simulink model "mcb_pmsm_foc_hall_f28035"  (R2021b)
settings: Solver=FixedStepDiscrete  StartTime=0.0  StopTime=8  RelTol=1e-3  EnableMultiTasking=on
InitFcn:
  | mcb_pmsm_foc_hall_f28035_data
values from neighbouring files (symbols this model uses):
  inverter = mcb_SetInverterParameters('BoostXL-DRV8305')    [mcb_pmsm_foc_dual_f28379d_data.m]    (also in mcb_pmsm_foc_dual_f28379d_datascript.m; mcb_pmsm_foc_f280049C_data.m; mcb_pmsm_foc_f28335_data.m = mcb_SetInverterParameters('DRV8312-C2-KIT'); mcb_pmsm_foc_hall_f28035_data.m = mcb_SetInverterParameters('DRV8312-C2-KIT'))
  PI_params = mcb.internal.SetControllerParameters(pmsm,inverter,PU_System,T_pwm,2*Ts,Ts_speed)    [mcb_pmsm_foc_dual_f28379d_data.m]    (also in mcb_pmsm_foc_dual_f28379d_datascript.m; mcb_pmsm_foc_f280049C_data.m = mcb.internal.SetControllerParameters(pmsm,inverter,PU_System; mcb_pmsm_foc_f28335_data.m = mcb.internal.SetControllerParameters(pmsm,inverter,PU_System; mcb_pmsm_foc_hall_f28035_data.m = mcb.internal.SetControllerParameters(pmsm,inverter,PU_System)
  pmsm = struct    [c28335_pmsmfoc_data.m]    (also in mcb_pmsm_foc_dual_f28379d_data.m = mcb_SetPMSMMotorParameters('Teknic2310P'); mcb_pmsm_foc_dual_f28379d_datascript.m = mcb_SetPMSMMotorParameters('Teknic2310P'); mcb_pmsm_foc_f280049C_data.m = mcb_SetPMSMMotorParameters('BLY171D'); mcb_pmsm_foc_f28335_data.m = mcb_SetPMSMMotorParameters('BLY171D'))
  target = mcb_SetProcessorDetails('F28379D',PWM_frequency)    [mcb_pmsm_foc_dual_f28379d_data.m]    (also in mcb_pmsm_foc_dual_f28379d_datascript.m; mcb_pmsm_foc_f280049C_data.m = mcb_SetProcessorDetails('F280049C',PWM_frequency); mcb_pmsm_foc_f28335_data.m = mcb_SetProcessorDetails('F28335',PWM_frequency); mcb_pmsm_foc_hall_f28035_data.m = mcb_SetProcessorDetails('F28035',PWM_frequency))
  Ts = 5e-8    (= 5e-08)    [DCDC_Buck_Param.m]    (also in mcb_c2000_open_loop_control_data.m = T_pwm; mcb_c2000_pmsm_offset_data.m = T_pwm; mcb_pmsm_foc_dual_f28379d_data.m = 5e-05; mcb_pmsm_foc_dual_f28379d_datascript.m = 5e-05)
  Ts_motor = T_pwm/2    (= 2.5e-05)    [mcb_pmsm_foc_dual_f28379d_data.m]    (also in mcb_pmsm_foc_dual_f28379d_datascript.m; mcb_pmsm_foc_f280049C_data.m; mcb_pmsm_foc_f28335_data.m; mcb_pmsm_foc_hall_f28035_data.m)
  Ts_simulink = T_pwm/2    (= 2.5e-05)    [mcb_pmsm_foc_dual_f28379d_data.m]    (also in mcb_pmsm_foc_dual_f28379d_datascript.m; mcb_pmsm_foc_f280049C_data.m; mcb_pmsm_foc_f28335_data.m; mcb_pmsm_foc_hall_f28035_data.m)
undefined symbols (not defined in the file or in its folder): Down, GPTRIP1SEL, GPTRIP2SEL, TZ1, TZ2, Up
libraries: simulink x16, idelinklib_common x15, mcbpositiondecoderlib x7, c2802xlib x5, mcbcontrolslib x3, c280xlib x3, hall_sensor_lib x3, c2803xlib x3, svdutilitieslib x2, demo_controls x1, c2000lib x1, mcbplantlib x1
(part 3 of 3)

== system mcb_pmsm_foc_hall_f28035/Embedded Processor/Hall Algorithm/Input Scaling/Read_Sensor (codegen)/Calculate Position from Hall/Atomic Hall Reading/Function-Call Subsystem1/Direction 0 Provides offset and counter values ==
  halls : Inport
  Action Port : ActionPort  ActionPortLabel=if(u1 == 1)
  Hall A falling : Subsystem  TreatAsAtomicUnit=on
  Hall A rising : Subsystem  TreatAsAtomicUnit=on
  Hall B falling : Subsystem  TreatAsAtomicUnit=on
  Hall B rising : Subsystem  TreatAsAtomicUnit=on
  Hall C falling : Subsystem  TreatAsAtomicUnit=on
  Hall C rising : Subsystem  TreatAsAtomicUnit=on
  Merge : Merge  Inputs=6
  Signal Conversion : SignalConversion  OverrideOpt=on
  Switch Case : SwitchCase  CaseConditions={1,2,3,4,5,6}  ShowDefaultCase=off
  counter : Outport
  wires:
  Signal Conversion/1 -> counter/1
  Hall B rising/1(counter) -> Merge/6
  Hall C rising/1(counter) -> Merge/5
  Hall A falling/1(counter) -> Merge/4
  Hall A rising/1(counter) -> Merge/3
  Hall C falling/1(counter) -> Merge/2
  Hall B falling/1(counter) -> Merge/1
  Merge/1 -> Signal Conversion/1
  Switch Case/4 -> Hall A falling/Action
  Switch Case/3 -> Hall A rising/Action
  Switch Case/1 -> Hall B falling/Action
  Switch Case/6 -> Hall B rising/Action
  Switch Case/5 -> Hall C rising/Action
  Switch Case/2 -> Hall C falling/Action
  halls/1 -> Switch Case/1

== system mcb_pmsm_foc_hall_f28035/Embedded Processor/Hall Algorithm/Input Scaling/Read_Sensor (codegen)/Calculate Position from Hall/Atomic Hall Reading/Function-Call Subsystem1/Direction 1 Provides offset and counter values ==
  halls : Inport
  Action Port : ActionPort  ActionPortLabel=else
  Hall A falling : Subsystem  TreatAsAtomicUnit=on
  Hall A rising : Subsystem  TreatAsAtomicUnit=on
  Hall B falling : Subsystem  TreatAsAtomicUnit=on
  Hall B rising : Subsystem  TreatAsAtomicUnit=on
  Hall C falling : Subsystem  TreatAsAtomicUnit=on
  Hall C rising : Subsystem  TreatAsAtomicUnit=on
  Merge : Merge  Inputs=6
  Switch Case : SwitchCase  CaseConditions={1,2,3,4,5,6}  ShowDefaultCase=off
  counter : Outport
  wires:
  Hall C rising/1(counter) -> Merge/6
  Hall A rising/1(counter) -> Merge/5
  Hall B falling/1(counter) -> Merge/4
  Hall B rising/1(counter) -> Merge/3
  Hall A falling/1(counter) -> Merge/2
  Hall C falling/1(counter) -> Merge/1
  Switch Case/4 -> Hall B falling/Action
  Switch Case/3 -> Hall B rising/Action
  Switch Case/1 -> Hall C falling/Action
  Switch Case/6 -> Hall C rising/Action
  Switch Case/5 -> Hall A rising/Action
  Switch Case/2 -> Hall A falling/Action
  halls/1 -> Switch Case/1
  Merge/1 -> counter/1

== system mcb_pmsm_foc_hall_f28035/Embedded Processor/Hall Algorithm/Input Scaling/Read_Sensor (codegen)/Calculate Position from Hall/Atomic Hall Reading/Function-Call Subsystem4/Direction 0 Provides offset and counter values ==
  halls : Inport
  In2 : Inport  Port=2
  Action Port : ActionPort  ActionPortLabel=if(u1 == 1)
  Hall A falling : Subsystem  TreatAsAtomicUnit=on
  Hall A rising : Subsystem  TreatAsAtomicUnit=on
  Hall B falling : Subsystem  TreatAsAtomicUnit=on
  Hall B rising : Subsystem  TreatAsAtomicUnit=on
  Hall C falling : Subsystem  TreatAsAtomicUnit=on
  Hall C rising : Subsystem  TreatAsAtomicUnit=on
  Merge : Merge  Inputs=6
  Signal Conversion : SignalConversion  OverrideOpt=on
  Switch Case : SwitchCase  CaseConditions={1,2,3,4,5,6}  ShowDefaultCase=off
  counter : Outport
  wires:
  In2/1 -> Hall B falling/1(In1), Hall C falling/1(In1), Hall A rising/1(In1), Hall A falling/1(In1), Hall C rising/1(In1), Hall B rising/1(In1)
  Signal Conversion/1 -> counter/1
  Hall B rising/1(counter) -> Merge/6
  Hall C rising/1(counter) -> Merge/5
  Hall A falling/1(counter) -> Merge/4
  Hall A rising/1(counter) -> Merge/3
  Hall C falling/1(counter) -> Merge/2
  Hall B falling/1(counter) -> Merge/1
  Merge/1 -> Signal Conversion/1
  Switch Case/4 -> Hall A falling/Action
  Switch Case/3 -> Hall A rising/Action
  Switch Case/1 -> Hall B falling/Action
  Switch Case/6 -> Hall B rising/Action
  Switch Case/5 -> Hall C rising/Action
  Switch Case/2 -> Hall C falling/Action
  halls/1 -> Switch Case/1

== system mcb_pmsm_foc_hall_f28035/Embedded Processor/Hall Algorithm/Input Scaling/Read_Sensor (codegen)/Calculate Position from Hall/Atomic Hall Reading/Function-Call Subsystem4/Direction 1 Provides offset and counter values ==
  In1 : Inport
  halls : Inport  Port=2
  Action Port : ActionPort  ActionPortLabel=else
  Hall A falling : Subsystem  TreatAsAtomicUnit=on
  Hall A rising : Subsystem  TreatAsAtomicUnit=on
  Hall B falling : Subsystem  TreatAsAtomicUnit=on
  Hall B rising : Subsystem  TreatAsAtomicUnit=on
  Hall C falling : Subsystem  TreatAsAtomicUnit=on
  Hall C rising : Subsystem  TreatAsAtomicUnit=on
  Merge : Merge  Inputs=6
  Switch Case : SwitchCase  CaseConditions={1,2,3,4,5,6}  ShowDefaultCase=off
  counter : Outport
  wires:
  In1/1 -> Hall C falling/1(In1), Hall A falling/1(In1), Hall B rising/1(In1), Hall B falling/1(In1), Hall A rising/1(In1), Hall C rising/1(In1)
  Hall C rising/1(counter) -> Merge/6
  Hall A rising/1(counter) -> Merge/5
  Hall B falling/1(counter) -> Merge/4
  Hall B rising/1(counter) -> Merge/3
  Hall A falling/1(counter) -> Merge/2
  Hall C falling/1(counter) -> Merge/1
  Switch Case/4 -> Hall B falling/Action
  Switch Case/3 -> Hall B rising/Action
  Switch Case/1 -> Hall C falling/Action
  Switch Case/6 -> Hall C rising/Action
  Switch Case/5 -> Hall A rising/Action
  Switch Case/2 -> Hall A falling/Action
  halls/1 -> Switch Case/1
  Merge/1 -> counter/1

== system mcb_pmsm_foc_hall_f28035/Embedded Processor/Hall Algorithm/Input Scaling/Read_Sensor (codegen)/Calculate Position from Hall/Atomic Hall Reading/Function-Call Subsystem/Integrity_Check/No_Integrity_issue ==
  Counter : Inport
  Action Port : ActionPort  ActionPortLabel=if(u1 == 0)
  Out1 : Outport
  wires:
  Counter/1 -> Out1/1

== system mcb_pmsm_foc_hall_f28035/Embedded Processor/Hall Algorithm/Input Scaling/Read_Sensor (codegen)/Calculate Position from Hall/Atomic Hall Reading/Function-Call Subsystem/Integrity_Check/Refresh_Halls ==
  Action Port : ActionPort  ActionPortLabel=else
  Bitwise AND : simulink/Logic and Bit Operations/Bitwise Operator  logicop=AND  UseBitMask=on  BitMask=hex2dec('07000000')  BitMaskRealWorld=Stored Integer
  Data Type Conversion : DataTypeConversion  OutDataTypeStr=uint32  ConvertRealWorld=Stored Integer (SI)
  Memory Copy3 : svdutilitieslib/Memory Copy  copyFrom=Specified source code symbol  copyFromAddressSource=Specify via dialog  copyFromAddress=hex2dec('00001000')  copyFromSrcCode=&GpioDataRegs.GPADAT.all  dataTypeFrom=uint32  dataDimensionFrom=1  useOffsetFrom=off  offsetFromSrc=Specify via dialog  offsetFrom=0  strideFrom=1  copyTo=Output port  copyToAddressSource=Specify via dialog  copyToAddress=hex2dec('00002000')  copyToSrcCode=myVariableDst  dataTypeTo=uint32  useOffsetTo=off  offsetToSrc=Specify via dialog  offsetTo=0  strideTo=1  sampleTime=-1  useInitValue=off  initValueSrc=Specify constant value  initValue=1  initValueSrcCode=myInitValueVariable  useAsMask=off  maskOperator=bitwise AND  useTermValue=off  termValue=1  isRealtimeEnabled=off  emitCCBeforeWrite=off  CCBeforeWrite=/* Custom Code Before Write*/  emitCCAfterWrite=off  CCAfterWrite=/* Custom Code After Write*/  useDMACopy=off  enableBlockingMode=off  blockPlatform=arduinoert
      settings: SourceProductBaseCode=ANDROID,ARDUINO,ML_ARDUINO,ECCORTEXA,ECCORTEXR,SC_BEAGLEBONE_BLUE,EC_FREEDOM_BOARD,EC_FRDM_K64F,INTEL_BLOCKSET,MICROBIT,NUCLEO,NVIDIA,PX4AUTOPILOTS,RASPPIIO,STMICRODIS,TIC2000,XILINX_BLOCKSET
  Shift Arithmetic : ArithShift  BitShiftNumber=24
  Out1 : Outport
  wires:
  Data Type Conversion/1 -> Out1/1
  Bitwise AND/1 -> Shift Arithmetic/1
  Shift Arithmetic/1 -> Data Type Conversion/1
  Memory Copy3/1 -> Bitwise AND/1

== system mcb_pmsm_foc_hall_f28035/Embedded Processor/Hall Algorithm/Input Scaling/Read_Sensor (codegen)/Calculate Position from Hall/Atomic Hall Reading/Function-Call Subsystem1/Direction 0 Provides offset and counter values/Hall A falling ==
  Action Port : ActionPort  ActionPortLabel=case [ 4 ]:
  ECap1Regs.TSCTR1 : idelinklib_common/Memory Copy  copyFrom=Specified source code symbol  copyFromAddressSource=Specify via dialog  copyFromAddress=hex2dec('00001000')  copyFromSrcCode=&ECap1Regs.TSCTR  dataTypeFrom=uint32  dataDimensionFrom=1  useOffsetFrom=off  offsetFromSrc=Specify via dialog  offsetFrom=0  strideFrom=1  copyTo=Output port  copyToAddressSource=Specify via dialog  copyToAddress=hex2dec('00002000')  copyToSrcCode=myVariableDst  dataTypeTo=uint32  useOffsetTo=off  offsetToSrc=Specify via dialog  offsetTo=0  strideTo=1  sampleTime=-1  useInitValue=off  initValueSrc=Specify constant value  initValue=1  initValueSrcCode=myInitValueVariable  useAsMask=off  maskOperator=bitwise AND  useTermValue=off  termValue=1  isRealtimeEnabled=off  emitCCBeforeWrite=off  CCBeforeWrite=/* Custom Code Before Write*/  emitCCAfterWrite=off  CCAfterWrite=/* Custom Code After Write*/  useDMACopy=off  enableBlockingMode=off
      settings: SourceProductBaseCode=ME
  counter : Outport
  wires:
  ECap1Regs.TSCTR1/1 -> counter/1

== system mcb_pmsm_foc_hall_f28035/Embedded Processor/Hall Algorithm/Input Scaling/Read_Sensor (codegen)/Calculate Position from Hall/Atomic Hall Reading/Function-Call Subsystem1/Direction 0 Provides offset and counter values/Hall A rising ==
  Action Port : ActionPort  ActionPortLabel=case [ 3 ]:
  ECap1Regs.TSCTR1 : idelinklib_common/Memory Copy  copyFrom=Specified source code symbol  copyFromAddressSource=Specify via dialog  copyFromAddress=hex2dec('00001000')  copyFromSrcCode=&ECap1Regs.TSCTR  dataTypeFrom=uint32  dataDimensionFrom=1  useOffsetFrom=off  offsetFromSrc=Specify via dialog  offsetFrom=0  strideFrom=1  copyTo=Output port  copyToAddressSource=Specify via dialog  copyToAddress=hex2dec('00002000')  copyToSrcCode=myVariableDst  dataTypeTo=uint32  useOffsetTo=off  offsetToSrc=Specify via dialog  offsetTo=0  strideTo=1  sampleTime=-1  useInitValue=off  initValueSrc=Specify constant value  initValue=1  initValueSrcCode=myInitValueVariable  useAsMask=off  maskOperator=bitwise AND  useTermValue=off  termValue=1  isRealtimeEnabled=off  emitCCBeforeWrite=off  CCBeforeWrite=/* Custom Code Before Write*/  emitCCAfterWrite=off  CCAfterWrite=/* Custom Code After Write*/  useDMACopy=off  enableBlockingMode=off
      settings: SourceProductBaseCode=ME
  counter : Outport
  wires:
  ECap1Regs.TSCTR1/1 -> counter/1

== system mcb_pmsm_foc_hall_f28035/Embedded Processor/Hall Algorithm/Input Scaling/Read_Sensor (codegen)/Calculate Position from Hall/Atomic Hall Reading/Function-Call Subsystem1/Direction 0 Provides offset and counter values/Hall B falling ==
  Action Port : ActionPort  ActionPortLabel=case [ 1 ]:
  Add : Sum  Inputs=-+  OutDataTypeStr=Inherit: Same as first input
  Data Store Read : DataStoreRead  DataStoreName=ECap1_counter_XINT1_latch  IndexOptions=Index vector (dialog)  Indices=1  OutputSizes=1
  ECap1Regs.TSCTR : idelinklib_common/Memory Copy  copyFrom=Specified source code symbol  copyFromAddressSource=Specify via dialog  copyFromAddress=hex2dec('00001000')  copyFromSrcCode=&ECap1Regs.TSCTR  dataTypeFrom=uint32  dataDimensionFrom=1  useOffsetFrom=off  offsetFromSrc=Specify via dialog  offsetFrom=0  strideFrom=1  copyTo=Output port  copyToAddressSource=Specify via dialog  copyToAddress=hex2dec('00002000')  copyToSrcCode=myVariableDst  dataTypeTo=uint32  useOffsetTo=off  offsetToSrc=Specify via dialog  offsetTo=0  strideTo=1  sampleTime=-1  useInitValue=off  initValueSrc=Specify constant value  initValue=1  initValueSrcCode=myInitValueVariable  useAsMask=off  maskOperator=bitwise AND  useTermValue=off  termValue=1  isRealtimeEnabled=off  emitCCBeforeWrite=off  CCBeforeWrite=/* Custom Code Before Write*/  emitCCAfterWrite=off  CCAfterWrite=/* Custom Code After Write*/  useDMACopy=off  enableBlockingMode=off
      settings: SourceProductBaseCode=ME
  counter : Outport
  wires:
  Add/1 -> counter/1
  ECap1Regs.TSCTR/1 -> Add/2
  Data Store Read/1 -> Add/1

== system mcb_pmsm_foc_hall_f28035/Embedded Processor/Hall Algorithm/Input Scaling/Read_Sensor (codegen)/Calculate Position from Hall/Atomic Hall Reading/Function-Call Subsystem1/Direction 0 Provides offset and counter values/Hall B rising ==
  Action Port : ActionPort  ActionPortLabel=case [ 6 ]:
  Add : Sum  Inputs=-+  OutDataTypeStr=Inherit: Same as first input
  Data Store Read : DataStoreRead  DataStoreName=ECap1_counter_XINT1_latch  IndexOptions=Index vector (dialog)  Indices=1  OutputSizes=1
  ECap1Regs.TSCTR : idelinklib_common/Memory Copy  copyFrom=Specified source code symbol  copyFromAddressSource=Specify via dialog  copyFromAddress=hex2dec('00001000')  copyFromSrcCode=&ECap1Regs.TSCTR  dataTypeFrom=uint32  dataDimensionFrom=1  useOffsetFrom=off  offsetFromSrc=Specify via dialog  offsetFrom=0  strideFrom=1  copyTo=Output port  copyToAddressSource=Specify via dialog  copyToAddress=hex2dec('00002000')  copyToSrcCode=myVariableDst  dataTypeTo=uint32  useOffsetTo=off  offsetToSrc=Specify via dialog  offsetTo=0  strideTo=1  sampleTime=-1  useInitValue=off  initValueSrc=Specify constant value  initValue=1  initValueSrcCode=myInitValueVariable  useAsMask=off  maskOperator=bitwise AND  useTermValue=off  termValue=1  isRealtimeEnabled=off  emitCCBeforeWrite=off  CCBeforeWrite=/* Custom Code Before Write*/  emitCCAfterWrite=off  CCAfterWrite=/* Custom Code After Write*/  useDMACopy=off  enableBlockingMode=off
      settings: SourceProductBaseCode=ME
  counter : Outport
  wires:
  ECap1Regs.TSCTR/1 -> Add/2
  Data Store Read/1 -> Add/1
  Add/1 -> counter/1

== system mcb_pmsm_foc_hall_f28035/Embedded Processor/Hall Algorithm/Input Scaling/Read_Sensor (codegen)/Calculate Position from Hall/Atomic Hall Reading/Function-Call Subsystem1/Direction 0 Provides offset and counter values/Hall C falling ==
  Action Port : ActionPort  ActionPortLabel=case [ 2 ]:
  Add : Sum  Inputs=-+  OutDataTypeStr=Inherit: Same as first input
  Data Store Read : DataStoreRead  DataStoreName=ECap1_counter_XINT2_latch  IndexOptions=Index vector (dialog)  Indices=1  OutputSizes=1
  ECap1Regs.TSCTR : idelinklib_common/Memory Copy  copyFrom=Specified source code symbol  copyFromAddressSource=Specify via dialog  copyFromAddress=hex2dec('00001000')  copyFromSrcCode=&ECap1Regs.TSCTR  dataTypeFrom=uint32  dataDimensionFrom=1  useOffsetFrom=off  offsetFromSrc=Specify via dialog  offsetFrom=0  strideFrom=1  copyTo=Output port  copyToAddressSource=Specify via dialog  copyToAddress=hex2dec('00002000')  copyToSrcCode=myVariableDst  dataTypeTo=uint32  useOffsetTo=off  offsetToSrc=Specify via dialog  offsetTo=0  strideTo=1  sampleTime=-1  useInitValue=off  initValueSrc=Specify constant value  initValue=1  initValueSrcCode=myInitValueVariable  useAsMask=off  maskOperator=bitwise AND  useTermValue=off  termValue=1  isRealtimeEnabled=off  emitCCBeforeWrite=off  CCBeforeWrite=/* Custom Code Before Write*/  emitCCAfterWrite=off  CCAfterWrite=/* Custom Code After Write*/  useDMACopy=off  enableBlockingMode=off
      settings: SourceProductBaseCode=ME
  counter : Outport
  wires:
  ECap1Regs.TSCTR/1 -> Add/2
  Data Store Read/1 -> Add/1
  Add/1 -> counter/1

== system mcb_pmsm_foc_hall_f28035/Embedded Processor/Hall Algorithm/Input Scaling/Read_Sensor (codegen)/Calculate Position from Hall/Atomic Hall Reading/Function-Call Subsystem1/Direction 0 Provides offset and counter values/Hall C rising ==
  Action Port : ActionPort  ActionPortLabel=case [ 5 ]:
  Add : Sum  Inputs=-+  OutDataTypeStr=Inherit: Same as first input
  Data Store Read : DataStoreRead  DataStoreName=ECap1_counter_XINT2_latch  IndexOptions=Index vector (dialog)  Indices=1  OutputSizes=1
  ECap1Regs.TSCTR : idelinklib_common/Memory Copy  copyFrom=Specified source code symbol  copyFromAddressSource=Specify via dialog  copyFromAddress=hex2dec('00001000')  copyFromSrcCode=&ECap1Regs.TSCTR  dataTypeFrom=uint32  dataDimensionFrom=1  useOffsetFrom=off  offsetFromSrc=Specify via dialog  offsetFrom=0  strideFrom=1  copyTo=Output port  copyToAddressSource=Specify via dialog  copyToAddress=hex2dec('00002000')  copyToSrcCode=myVariableDst  dataTypeTo=uint32  useOffsetTo=off  offsetToSrc=Specify via dialog  offsetTo=0  strideTo=1  sampleTime=-1  useInitValue=off  initValueSrc=Specify constant value  initValue=1  initValueSrcCode=myInitValueVariable  useAsMask=off  maskOperator=bitwise AND  useTermValue=off  termValue=1  isRealtimeEnabled=off  emitCCBeforeWrite=off  CCBeforeWrite=/* Custom Code Before Write*/  emitCCAfterWrite=off  CCAfterWrite=/* Custom Code After Write*/  useDMACopy=off  enableBlockingMode=off
      settings: SourceProductBaseCode=ME
  counter : Outport
  wires:
  ECap1Regs.TSCTR/1 -> Add/2
  Data Store Read/1 -> Add/1
  Add/1 -> counter/1

== system mcb_pmsm_foc_hall_f28035/Embedded Processor/Hall Algorithm/Input Scaling/Read_Sensor (codegen)/Calculate Position from Hall/Atomic Hall Reading/Function-Call Subsystem1/Direction 1 Provides offset and counter values/Hall A falling ==
  Action Port : ActionPort  ActionPortLabel=case [ 2 ]:
  ECap1Regs.TSCTR1 : idelinklib_common/Memory Copy  copyFrom=Specified source code symbol  copyFromAddressSource=Specify via dialog  copyFromAddress=hex2dec('00001000')  copyFromSrcCode=&ECap1Regs.TSCTR  dataTypeFrom=uint32  dataDimensionFrom=1  useOffsetFrom=off  offsetFromSrc=Specify via dialog  offsetFrom=0  strideFrom=1  copyTo=Output port  copyToAddressSource=Specify via dialog  copyToAddress=hex2dec('00002000')  copyToSrcCode=myVariableDst  dataTypeTo=uint32  useOffsetTo=off  offsetToSrc=Specify via dialog  offsetTo=0  strideTo=1  sampleTime=-1  useInitValue=off  initValueSrc=Specify constant value  initValue=1  initValueSrcCode=myInitValueVariable  useAsMask=off  maskOperator=bitwise AND  useTermValue=off  termValue=1  isRealtimeEnabled=off  emitCCBeforeWrite=off  CCBeforeWrite=/* Custom Code Before Write*/  emitCCAfterWrite=off  CCAfterWrite=/* Custom Code After Write*/  useDMACopy=off  enableBlockingMode=off
      settings: SourceProductBaseCode=ME
  counter : Outport
  wires:
  ECap1Regs.TSCTR1/1 -> counter/1

== system mcb_pmsm_foc_hall_f28035/Embedded Processor/Hall Algorithm/Input Scaling/Read_Sensor (codegen)/Calculate Position from Hall/Atomic Hall Reading/Function-Call Subsystem1/Direction 1 Provides offset and counter values/Hall A rising ==
  Action Port : ActionPort  ActionPortLabel=case [ 5 ]:
  ECap1Regs.TSCTR1 : idelinklib_common/Memory Copy  copyFrom=Specified source code symbol  copyFromAddressSource=Specify via dialog  copyFromAddress=hex2dec('00001000')  copyFromSrcCode=&ECap1Regs.TSCTR  dataTypeFrom=uint32  dataDimensionFrom=1  useOffsetFrom=off  offsetFromSrc=Specify via dialog  offsetFrom=0  strideFrom=1  copyTo=Output port  copyToAddressSource=Specify via dialog  copyToAddress=hex2dec('00002000')  copyToSrcCode=myVariableDst  dataTypeTo=uint32  useOffsetTo=off  offsetToSrc=Specify via dialog  offsetTo=0  strideTo=1  sampleTime=-1  useInitValue=off  initValueSrc=Specify constant value  initValue=1  initValueSrcCode=myInitValueVariable  useAsMask=off  maskOperator=bitwise AND  useTermValue=off  termValue=1  isRealtimeEnabled=off  emitCCBeforeWrite=off  CCBeforeWrite=/* Custom Code Before Write*/  emitCCAfterWrite=off  CCAfterWrite=/* Custom Code After Write*/  useDMACopy=off  enableBlockingMode=off
      settings: SourceProductBaseCode=ME
  counter : Outport
  wires:
  ECap1Regs.TSCTR1/1 -> counter/1

== system mcb_pmsm_foc_hall_f28035/Embedded Processor/Hall Algorithm/Input Scaling/Read_Sensor (codegen)/Calculate Position from Hall/Atomic Hall Reading/Function-Call Subsystem1/Direction 1 Provides offset and counter values/Hall B falling ==
  Action Port : ActionPort  ActionPortLabel=case [ 4 ]:
  Add : Sum  Inputs=+-  OutDataTypeStr=Inherit: Same as first input
  Data Store Read : DataStoreRead  DataStoreName=ECap1_counter_XINT1_latch  IndexOptions=Index vector (dialog)  Indices=1  OutputSizes=1
  ECap1Regs.TSCTR : idelinklib_common/Memory Copy  copyFrom=Specified source code symbol  copyFromAddressSource=Specify via dialog  copyFromAddress=hex2dec('00001000')  copyFromSrcCode=&ECap1Regs.TSCTR  dataTypeFrom=uint32  dataDimensionFrom=1  useOffsetFrom=off  offsetFromSrc=Specify via dialog  offsetFrom=0  strideFrom=1  copyTo=Output port  copyToAddressSource=Specify via dialog  copyToAddress=hex2dec('00002000')  copyToSrcCode=myVariableDst  dataTypeTo=uint32  useOffsetTo=off  offsetToSrc=Specify via dialog  offsetTo=0  strideTo=1  sampleTime=-1  useInitValue=off  initValueSrc=Specify constant value  initValue=1  initValueSrcCode=myInitValueVariable  useAsMask=off  maskOperator=bitwise AND  useTermValue=off  termValue=1  isRealtimeEnabled=off  emitCCBeforeWrite=off  CCBeforeWrite=/* Custom Code Before Write*/  emitCCAfterWrite=off  CCAfterWrite=/* Custom Code After Write*/  useDMACopy=off  enableBlockingMode=off
      settings: SourceProductBaseCode=ME
  counter : Outport
  wires:
  ECap1Regs.TSCTR/1 -> Add/1
  Data Store Read/1 -> Add/2
  Add/1 -> counter/1

== system mcb_pmsm_foc_hall_f28035/Embedded Processor/Hall Algorithm/Input Scaling/Read_Sensor (codegen)/Calculate Position from Hall/Atomic Hall Reading/Function-Call Subsystem1/Direction 1 Provides offset and counter values/Hall B rising ==
  Action Port : ActionPort  ActionPortLabel=case [ 3 ]:
  Add : Sum  Inputs=-+  OutDataTypeStr=Inherit: Same as first input
  Data Store Read : DataStoreRead  DataStoreName=ECap1_counter_XINT1_latch  IndexOptions=Index vector (dialog)  Indices=1  OutputSizes=1
  ECap1Regs.TSCTR : idelinklib_common/Memory Copy  copyFrom=Specified source code symbol  copyFromAddressSource=Specify via dialog  copyFromAddress=hex2dec('00001000')  copyFromSrcCode=&ECap1Regs.TSCTR  dataTypeFrom=uint32  dataDimensionFrom=1  useOffsetFrom=off  offsetFromSrc=Specify via dialog  offsetFrom=0  strideFrom=1  copyTo=Output port  copyToAddressSource=Specify via dialog  copyToAddress=hex2dec('00002000')  copyToSrcCode=myVariableDst  dataTypeTo=uint32  useOffsetTo=off  offsetToSrc=Specify via dialog  offsetTo=0  strideTo=1  sampleTime=-1  useInitValue=off  initValueSrc=Specify constant value  initValue=1  initValueSrcCode=myInitValueVariable  useAsMask=off  maskOperator=bitwise AND  useTermValue=off  termValue=1  isRealtimeEnabled=off  emitCCBeforeWrite=off  CCBeforeWrite=/* Custom Code Before Write*/  emitCCAfterWrite=off  CCAfterWrite=/* Custom Code After Write*/  useDMACopy=off  enableBlockingMode=off
      settings: SourceProductBaseCode=ME
  counter : Outport
  wires:
  ECap1Regs.TSCTR/1 -> Add/2
  Data Store Read/1 -> Add/1
  Add/1 -> counter/1

== system mcb_pmsm_foc_hall_f28035/Embedded Processor/Hall Algorithm/Input Scaling/Read_Sensor (codegen)/Calculate Position from Hall/Atomic Hall Reading/Function-Call Subsystem1/Direction 1 Provides offset and counter values/Hall C falling ==
  Action Port : ActionPort  ActionPortLabel=case [ 1 ]:
  Add : Sum  Inputs=-+  OutDataTypeStr=Inherit: Same as first input
  Data Store Read : DataStoreRead  DataStoreName=ECap1_counter_XINT2_latch  IndexOptions=Index vector (dialog)  Indices=1  OutputSizes=1
  ECap1Regs.TSCTR : idelinklib_common/Memory Copy  copyFrom=Specified source code symbol  copyFromAddressSource=Specify via dialog  copyFromAddress=hex2dec('00001000')  copyFromSrcCode=&ECap1Regs.TSCTR  dataTypeFrom=uint32  dataDimensionFrom=1  useOffsetFrom=off  offsetFromSrc=Specify via dialog  offsetFrom=0  strideFrom=1  copyTo=Output port  copyToAddressSource=Specify via dialog  copyToAddress=hex2dec('00002000')  copyToSrcCode=myVariableDst  dataTypeTo=uint32  useOffsetTo=off  offsetToSrc=Specify via dialog  offsetTo=0  strideTo=1  sampleTime=-1  useInitValue=off  initValueSrc=Specify constant value  initValue=1  initValueSrcCode=myInitValueVariable  useAsMask=off  maskOperator=bitwise AND  useTermValue=off  termValue=1  isRealtimeEnabled=off  emitCCBeforeWrite=off  CCBeforeWrite=/* Custom Code Before Write*/  emitCCAfterWrite=off  CCAfterWrite=/* Custom Code After Write*/  useDMACopy=off  enableBlockingMode=off
      settings: SourceProductBaseCode=ME
  counter : Outport
  wires:
  Data Store Read/1 -> Add/1
  ECap1Regs.TSCTR/1 -> Add/2
  Add/1 -> counter/1

== system mcb_pmsm_foc_hall_f28035/Embedded Processor/Hall Algorithm/Input Scaling/Read_Sensor (codegen)/Calculate Position from Hall/Atomic Hall Reading/Function-Call Subsystem1/Direction 1 Provides offset and counter values/Hall C rising ==
  Action Port : ActionPort  ActionPortLabel=case [ 6 ]:
  Add : Sum  Inputs=-+  OutDataTypeStr=Inherit: Same as first input
  Data Store Read : DataStoreRead  DataStoreName=ECap1_counter_XINT2_latch  IndexOptions=Index vector (dialog)  Indices=1  OutputSizes=1
  ECap1Regs.TSCTR : idelinklib_common/Memory Copy  copyFrom=Specified source code symbol  copyFromAddressSource=Specify via dialog  copyFromAddress=hex2dec('00001000')  copyFromSrcCode=&ECap1Regs.TSCTR  dataTypeFrom=uint32  dataDimensionFrom=1  useOffsetFrom=off  offsetFromSrc=Specify via dialog  offsetFrom=0  strideFrom=1  copyTo=Output port  copyToAddressSource=Specify via dialog  copyToAddress=hex2dec('00002000')  copyToSrcCode=myVariableDst  dataTypeTo=uint32  useOffsetTo=off  offsetToSrc=Specify via dialog  offsetTo=0  strideTo=1  sampleTime=-1  useInitValue=off  initValueSrc=Specify constant value  initValue=1  initValueSrcCode=myInitValueVariable  useAsMask=off  maskOperator=bitwise AND  useTermValue=off  termValue=1  isRealtimeEnabled=off  emitCCBeforeWrite=off  CCBeforeWrite=/* Custom Code Before Write*/  emitCCAfterWrite=off  CCAfterWrite=/* Custom Code After Write*/  useDMACopy=off  enableBlockingMode=off
      settings: SourceProductBaseCode=ME
  counter : Outport
  wires:
  Data Store Read/1 -> Add/1
  ECap1Regs.TSCTR/1 -> Add/2
  Add/1 -> counter/1

== system mcb_pmsm_foc_hall_f28035/Embedded Processor/Hall Algorithm/Input Scaling/Read_Sensor (codegen)/Calculate Position from Hall/Atomic Hall Reading/Function-Call Subsystem4/Direction 0 Provides offset and counter values/Hall A falling ==
  In1 : Inport
  Action Port : ActionPort  ActionPortLabel=case [ 4 ]:
  counter : Outport
  wires:
  In1/1 -> counter/1

== system mcb_pmsm_foc_hall_f28035/Embedded Processor/Hall Algorithm/Input Scaling/Read_Sensor (codegen)/Calculate Position from Hall/Atomic Hall Reading/Function-Call Subsystem4/Direction 0 Provides offset and counter values/Hall A rising ==
  In1 : Inport
  Action Port : ActionPort  ActionPortLabel=case [ 3 ]:
  counter : Outport
  wires:
  In1/1 -> counter/1

== system mcb_pmsm_foc_hall_f28035/Embedded Processor/Hall Algorithm/Input Scaling/Read_Sensor (codegen)/Calculate Position from Hall/Atomic Hall Reading/Function-Call Subsystem4/Direction 0 Provides offset and counter values/Hall B falling ==
  In1 : Inport
  Action Port : ActionPort  ActionPortLabel=case [ 1 ]:
  Add : Sum  Inputs=-+  OutDataTypeStr=Inherit: Same as first input
  Data Store Read : DataStoreRead  DataStoreName=ECap1_counter_XINT1_latch  IndexOptions=Index vector (dialog)  Indices=1  OutputSizes=1
  counter : Outport
  wires:
  Add/1 -> counter/1
  In1/1 -> Add/2
  Data Store Read/1 -> Add/1

== system mcb_pmsm_foc_hall_f28035/Embedded Processor/Hall Algorithm/Input Scaling/Read_Sensor (codegen)/Calculate Position from Hall/Atomic Hall Reading/Function-Call Subsystem4/Direction 0 Provides offset and counter values/Hall B rising ==
  In1 : Inport
  Action Port : ActionPort  ActionPortLabel=case [ 6 ]:
  Add : Sum  Inputs=-+  OutDataTypeStr=Inherit: Same as first input
  Data Store Read : DataStoreRead  DataStoreName=ECap1_counter_XINT1_latch  IndexOptions=Index vector (dialog)  Indices=1  OutputSizes=1
  counter : Outport
  wires:
  In1/1 -> Add/2
  Data Store Read/1 -> Add/1
  Add/1 -> counter/1

== system mcb_pmsm_foc_hall_f28035/Embedded Processor/Hall Algorithm/Input Scaling/Read_Sensor (codegen)/Calculate Position from Hall/Atomic Hall Reading/Function-Call Subsystem4/Direction 0 Provides offset and counter values/Hall C falling ==
  In1 : Inport
  Action Port : ActionPort  ActionPortLabel=case [ 2 ]:
  Add : Sum  Inputs=-+  OutDataTypeStr=Inherit: Same as first input
  Data Store Read : DataStoreRead  DataStoreName=ECap1_counter_XINT2_latch  IndexOptions=Index vector (dialog)  Indices=1  OutputSizes=1
  counter : Outport
  wires:
  In1/1 -> Add/2
  Data Store Read/1 -> Add/1
  Add/1 -> counter/1

== system mcb_pmsm_foc_hall_f28035/Embedded Processor/Hall Algorithm/Input Scaling/Read_Sensor (codegen)/Calculate Position from Hall/Atomic Hall Reading/Function-Call Subsystem4/Direction 0 Provides offset and counter values/Hall C rising ==
  In1 : Inport
  Action Port : ActionPort  ActionPortLabel=case [ 5 ]:
  Add : Sum  Inputs=-+  OutDataTypeStr=Inherit: Same as first input
  Data Store Read : DataStoreRead  DataStoreName=ECap1_counter_XINT2_latch  IndexOptions=Index vector (dialog)  Indices=1  OutputSizes=1
  counter : Outport
  wires:
  In1/1 -> Add/2
  Data Store Read/1 -> Add/1
  Add/1 -> counter/1

== system mcb_pmsm_foc_hall_f28035/Embedded Processor/Hall Algorithm/Input Scaling/Read_Sensor (codegen)/Calculate Position from Hall/Atomic Hall Reading/Function-Call Subsystem4/Direction 1 Provides offset and counter values/Hall A falling ==
  In1 : Inport
  Action Port : ActionPort  ActionPortLabel=case [ 2 ]:
  counter : Outport
  wires:
  In1/1 -> counter/1

== system mcb_pmsm_foc_hall_f28035/Embedded Processor/Hall Algorithm/Input Scaling/Read_Sensor (codegen)/Calculate Position from Hall/Atomic Hall Reading/Function-Call Subsystem4/Direction 1 Provides offset and counter values/Hall A rising ==
  In1 : Inport
  Action Port : ActionPort  ActionPortLabel=case [ 5 ]:
  counter : Outport
  wires:
  In1/1 -> counter/1

== system mcb_pmsm_foc_hall_f28035/Embedded Processor/Hall Algorithm/Input Scaling/Read_Sensor (codegen)/Calculate Position from Hall/Atomic Hall Reading/Function-Call Subsystem4/Direction 1 Provides offset and counter values/Hall B falling ==
  In1 : Inport
  Action Port : ActionPort  ActionPortLabel=case [ 4 ]:
  Add : Sum  Inputs=+-  OutDataTypeStr=Inherit: Same as first input
  Data Store Read : DataStoreRead  DataStoreName=ECap1_counter_XINT1_latch  IndexOptions=Index vector (dialog)  Indices=1  OutputSizes=1
  counter : Outport
  wires:
  In1/1 -> Add/1
  Data Store Read/1 -> Add/2
  Add/1 -> counter/1

== system mcb_pmsm_foc_hall_f28035/Embedded Processor/Hall Algorithm/Input Scaling/Read_Sensor (codegen)/Calculate Position from Hall/Atomic Hall Reading/Function-Call Subsystem4/Direction 1 Provides offset and counter values/Hall B rising ==
  In1 : Inport
  Action Port : ActionPort  ActionPortLabel=case [ 3 ]:
  Add : Sum  Inputs=-+  OutDataTypeStr=Inherit: Same as first input
  Data Store Read : DataStoreRead  DataStoreName=ECap1_counter_XINT1_latch  IndexOptions=Index vector (dialog)  Indices=1  OutputSizes=1
  counter : Outport
  wires:
  In1/1 -> Add/2
  Data Store Read/1 -> Add/1
  Add/1 -> counter/1

== system mcb_pmsm_foc_hall_f28035/Embedded Processor/Hall Algorithm/Input Scaling/Read_Sensor (codegen)/Calculate Position from Hall/Atomic Hall Reading/Function-Call Subsystem4/Direction 1 Provides offset and counter values/Hall C falling ==
  In1 : Inport
  Action Port : ActionPort  ActionPortLabel=case [ 1 ]:
  Add : Sum  Inputs=-+  OutDataTypeStr=Inherit: Same as first input
  Data Store Read : DataStoreRead  DataStoreName=ECap1_counter_XINT2_latch  IndexOptions=Index vector (dialog)  Indices=1  OutputSizes=1
  counter : Outport
  wires:
  Data Store Read/1 -> Add/1
  In1/1 -> Add/2
  Add/1 -> counter/1

== system mcb_pmsm_foc_hall_f28035/Embedded Processor/Hall Algorithm/Input Scaling/Read_Sensor (codegen)/Calculate Position from Hall/Atomic Hall Reading/Function-Call Subsystem4/Direction 1 Provides offset and counter values/Hall C rising ==
  In1 : Inport
  Action Port : ActionPort  ActionPortLabel=case [ 6 ]:
  Add : Sum  Inputs=-+  OutDataTypeStr=Inherit: Same as first input
  Data Store Read : DataStoreRead  DataStoreName=ECap1_counter_XINT2_latch  IndexOptions=Index vector (dialog)  Indices=1  OutputSizes=1
  counter : Outport
  wires:
  Data Store Read/1 -> Add/1
  In1/1 -> Add/2
  Add/1 -> counter/1
